simulink model "Linear_Moving_Setpoint_Poly_Setting"  (R2020b)
settings: Solver=VariableStepAuto  StartTime=0.0  StopTime=t_sim  RelTol=1e-9
undefined symbols (not defined in the file): A1a_sim, B1a_sim, C1_polyset, des_traj_handle, M1_sim, M2_sim, x1a_0
settings Model: Creator=domin  LastModifiedBy=domin

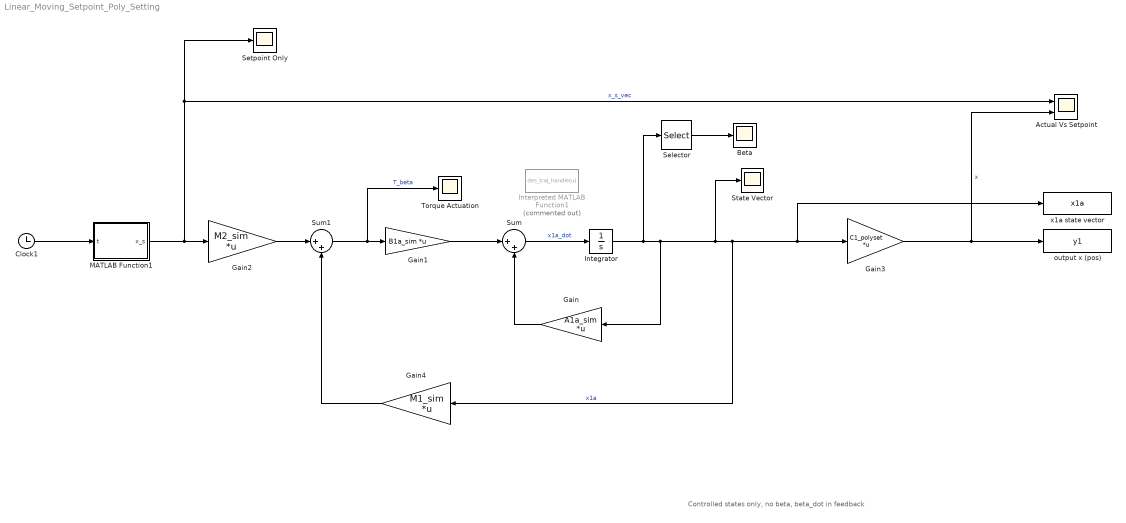
== system Linear_Moving_Setpoint_Poly_Setting ==
  note: Controlled states only, no beta, beta_dot in feedback
  Actual Vs Setpoint : Scope  NumInputPorts=2
  Beta : Scope
  Clock1 : Clock
  Gain : Gain  Gain=A1a_sim  Multiplication=Matrix(K*u)
  Gain1 : Gain  Gain=B1a_sim  Multiplication=Matrix(K*u)
  Gain2 : Gain  Gain=M2_sim  Multiplication=Matrix(K*u)
  Gain3 : Gain  Gain=C1_polyset  Multiplication=Matrix(K*u)
  Gain4 : Gain  Gain=M1_sim  Multiplication=Matrix(K*u)
  Integrator : Integrator  InitialCondition=x1a_0
  Interpreted MATLAB Function1 : MATLABFcn  Commented=on  MATLABFcn=des_traj_handle(u)
  MATLAB Function1 : MATLAB Function  TreatAsAtomicUnit=on
  Selector : Selector  InputPortWidth=5  IndexOptions=Index vector (dialog)  Indices=[4]  OutputSizes=1
  Setpoint Only : Scope
  State Vector : Scope
  Sum : Sum  Inputs=|++
  Sum1 : Sum  Inputs=|++
  Torque Actuation : Scope
  output x (pos) : ToWorkspace  VariableName=y1  SampleTime=-1
  x1a state vector : ToWorkspace  VariableName=x1a  SampleTime=-1
  wires:
  Gain3/1 -> Actual Vs Setpoint/2, output x (pos)/1  "x"
  Selector/1 -> Beta/1
  Gain1/1 -> Sum/1
  Gain/1 -> Sum/2
  MATLAB Function1/1(x_s) -> Setpoint Only/1, Actual Vs Setpoint/1, Gain2/1  "x_s_vec"
  Clock1/1 -> MATLAB Function1/1(t)
  Sum1/1 -> Torque Actuation/1, Gain1/1  "T_beta"
  Integrator/1 -> State Vector/1, x1a state vector/1, Gain3/1, Gain4/1, Gain/1, Selector/1  "x1a"
  Gain2/1 -> Sum1/1
  Sum/1 -> Integrator/1  "x1a_dot"
  Gain4/1 -> Sum1/2

== matlab function Linear_Moving_Setpoint_Poly_Setting/MATLAB Function1 ==
  data: t input; x_s output
function x_s = fcn(t)

x_s = [(pi.*-7.5e+1)./(pi.^2./4.0+2.5e+1./1.6e+1)-...
    (cos((t.*pi)./2.0).*3.0e+2)./pi+3.0e+2./pi+(exp(t.*(-5.0./4.0)).*...
    (sin((t.*pi)./2.0).*(5.0./4.0)+(pi.*cos((t.*pi)./2.0))./2.0).*1.5e+2)./...
    (pi.^2./4.0+2.5e+1./1.6e+1);...
    ...
    sin((t.*pi)./2.0).*(exp(t.*(-5.0./4.0))-1.0).*...
    -1.5e+2;...
    ...
    exp(t.*(-5.0./4.0)).*sin((t.*pi)./2.0).*(3.75e+2./2.0)-pi.*...
    cos((t.*pi)./2.0).*(exp(t.*(-5.0./4.0))-1.0).*7.5e+1];
